simulink model "slidingSimulation"  (R2017a)
settings: Solver=VariableStepAuto  StartTime=0.0  StopTime=10.0  RelTol=1e-3
values from neighbouring files (symbols this model uses):
  leaderAcceleration = 1    [sliding.m]
undefined symbols (not defined in the file or in its folder): chi, K, Ldes, slidingFunction, wn
settings Model: Creator=tlara  LastModifiedBy=tlara

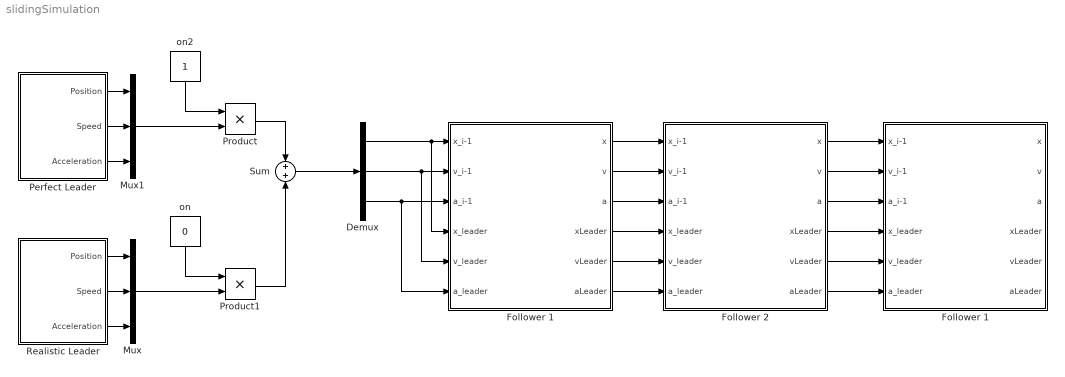
== system slidingSimulation ==
  Demux : Demux  Outputs=3
  Follower 1 : Subsystem
  "Follower 1 " : Subsystem
  Follower 2 : Subsystem
  Mux : Mux  Inputs=3
  Mux1 : Mux  Inputs=3
  Perfect Leader : Subsystem
  Product : Product
  Product1 : Product
  Realistic Leader : Subsystem
  Sum : Sum
  on : Constant  Value=0
  on2 : Constant
  wires:
  "Follower 1 "/1(x) -> Follower 2/1("x_i-1 ")
  "Follower 1 "/2(v) -> Follower 2/2(v_i-1)
  "Follower 1 "/3(a) -> Follower 2/3(a_i-1)
  "Follower 1 "/4(xLeader) -> Follower 2/4(x_leader)
  "Follower 1 "/5("vLeader ") -> Follower 2/5(v_leader)
  "Follower 1 "/6(aLeader) -> Follower 2/6(a_leader)
  Follower 2/6(aLeader) -> Follower 1/6(a_leader)
  Follower 2/5("vLeader ") -> Follower 1/5(v_leader)
  Follower 2/4(xLeader) -> Follower 1/4(x_leader)
  Follower 2/3(a) -> Follower 1/3(a_i-1)
  Follower 2/1(x) -> Follower 1/1("x_i-1 ")
  Follower 2/2(v) -> Follower 1/2(v_i-1)
  Realistic Leader/1(Position) -> Mux/1
  Realistic Leader/2(Speed) -> Mux/2
  Realistic Leader/3(Acceleration) -> Mux/3
  Perfect Leader/1(Position) -> Mux1/1
  Perfect Leader/2(Speed) -> Mux1/2
  Perfect Leader/3(Acceleration) -> Mux1/3
  Mux1/1 -> Product/2
  Mux/1 -> Product1/2
  on/1 -> Product1/1
  on2/1 -> Product/1
  Product/1 -> Sum/1
  Product1/1 -> Sum/2
  Sum/1 -> Demux/1
  Demux/3 -> "Follower 1 "/6(a_leader), "Follower 1 "/3(a_i-1)
  Demux/2 -> "Follower 1 "/5(v_leader), "Follower 1 "/2(v_i-1)
  Demux/1 -> "Follower 1 "/4(x_leader), "Follower 1 "/1("x_i-1 ")

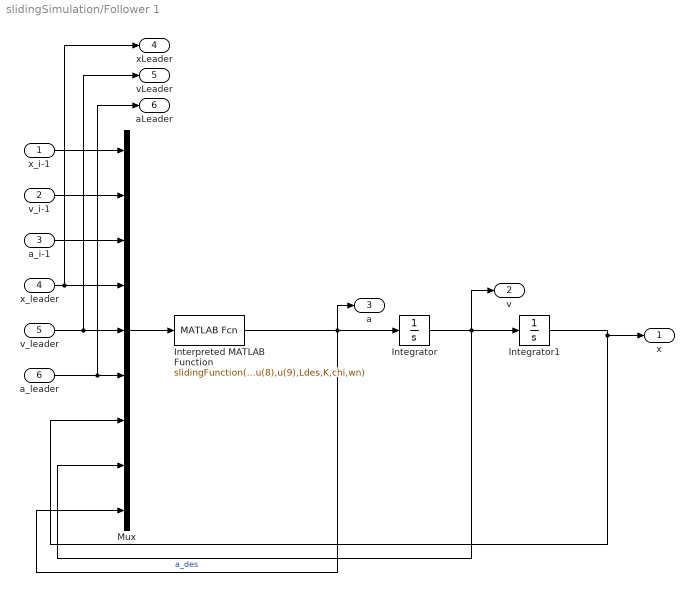
== system slidingSimulation/Follower 1 ==
  "x_i-1 " : Inport
  v_i-1 : Inport  Port=2
  a_i-1 : Inport  Port=3
  x_leader : Inport  Port=4
  v_leader : Inport  Port=5
  a_leader : Inport  Port=6
  Integrator : Integrator
  Integrator1 : Integrator
  Interpreted MATLAB Function : MATLABFcn  MATLABFcn=slidingFunction(u(1),u(2),u(3),u(4),u(5),u(6),u(7),u(8),u(9),Ldes,K,chi,wn)  OutputDimensions=1
  Mux : Mux  Inputs=9
  x : Outport
  v : Outport  Port=2
  a : Outport  Port=3
  xLeader : Outport  Port=4
  "vLeader " : Outport  Port=5
  aLeader : Outport  Port=6
  wires:
  Interpreted MATLAB Function/1 -> a/1, Mux/9, Integrator/1  "a_des"
  "x_i-1 "/1 -> Mux/1
  v_i-1/1 -> Mux/2
  a_i-1/1 -> Mux/3
  x_leader/1 -> xLeader/1, Mux/4
  v_leader/1 -> "vLeader "/1, Mux/5
  a_leader/1 -> aLeader/1, Mux/6
  Integrator1/1 -> Mux/7, x/1
  Mux/1 -> Interpreted MATLAB Function/1
  Integrator/1 -> v/1, Integrator1/1, Mux/8

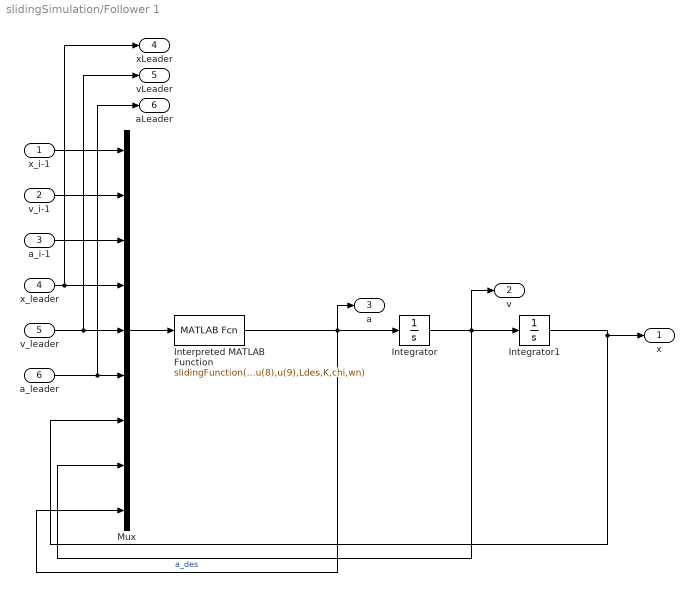
== system slidingSimulation/Follower 1  ==
  "x_i-1 " : Inport
  v_i-1 : Inport  Port=2
  a_i-1 : Inport  Port=3
  x_leader : Inport  Port=4
  v_leader : Inport  Port=5
  a_leader : Inport  Port=6
  Integrator : Integrator
  Integrator1 : Integrator
  Interpreted MATLAB Function : MATLABFcn  MATLABFcn=slidingFunction(u(1),u(2),u(3),u(4),u(5),u(6),u(7),u(8),u(9),Ldes,K,chi,wn)  OutputDimensions=1
  Mux : Mux  Inputs=9
  x : Outport
  v : Outport  Port=2
  a : Outport  Port=3
  xLeader : Outport  Port=4
  "vLeader " : Outport  Port=5
  aLeader : Outport  Port=6
  wires:
  Interpreted MATLAB Function/1 -> a/1, Mux/9, Integrator/1  "a_des"
  "x_i-1 "/1 -> Mux/1
  v_i-1/1 -> Mux/2
  a_i-1/1 -> Mux/3
  x_leader/1 -> xLeader/1, Mux/4
  v_leader/1 -> "vLeader "/1, Mux/5
  a_leader/1 -> aLeader/1, Mux/6
  Integrator1/1 -> Mux/7, x/1
  Mux/1 -> Interpreted MATLAB Function/1
  Integrator/1 -> v/1, Integrator1/1, Mux/8

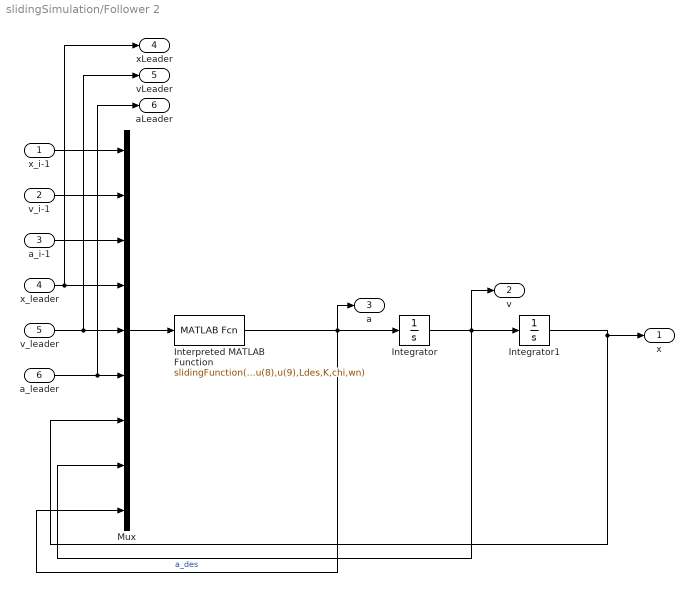
== system slidingSimulation/Follower 2 ==
  "x_i-1 " : Inport
  v_i-1 : Inport  Port=2
  a_i-1 : Inport  Port=3
  x_leader : Inport  Port=4
  v_leader : Inport  Port=5
  a_leader : Inport  Port=6
  Integrator : Integrator
  Integrator1 : Integrator
  Interpreted MATLAB Function : MATLABFcn  MATLABFcn=slidingFunction(u(1),u(2),u(3),u(4),u(5),u(6),u(7),u(8),u(9),Ldes,K,chi,wn)  OutputDimensions=1
  Mux : Mux  Inputs=9
  x : Outport
  v : Outport  Port=2
  a : Outport  Port=3
  xLeader : Outport  Port=4
  "vLeader " : Outport  Port=5
  aLeader : Outport  Port=6
  wires:
  Interpreted MATLAB Function/1 -> a/1, Mux/9, Integrator/1  "a_des"
  "x_i-1 "/1 -> Mux/1
  v_i-1/1 -> Mux/2
  a_i-1/1 -> Mux/3
  x_leader/1 -> xLeader/1, Mux/4
  v_leader/1 -> "vLeader "/1, Mux/5
  a_leader/1 -> aLeader/1, Mux/6
  Integrator1/1 -> Mux/7, x/1
  Mux/1 -> Interpreted MATLAB Function/1
  Integrator/1 -> v/1, Integrator1/1, Mux/8

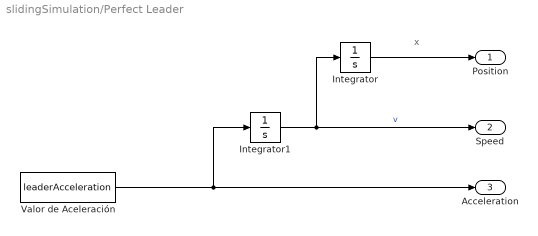
== system slidingSimulation/Perfect Leader ==
  note: x
  Integrator : Integrator
  Integrator1 : Integrator
  Valor de Aceleración : Constant  Value=leaderAcceleration
  Position : Outport
  Speed : Outport  Port=2
  Acceleration : Outport  Port=3
  wires:
  Integrator/1 -> Position/1
  Valor de Aceleración/1 -> Integrator1/1, Acceleration/1
  Integrator1/1 -> Integrator/1, Speed/1  "v"

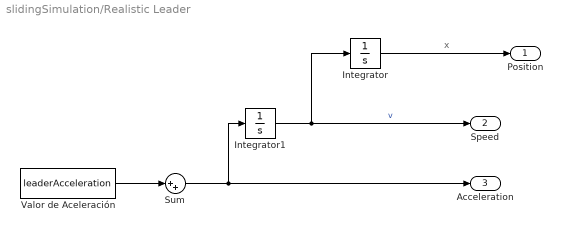
== system slidingSimulation/Realistic Leader ==
  note: x
  Integrator : Integrator
  Integrator1 : Integrator
  Sum : Sum  Inputs=|++
  Valor de Aceleración : Constant  Value=leaderAcceleration
  Position : Outport
  Speed : Outport  Port=2
  Acceleration : Outport  Port=3
  wires:
  Integrator/1 -> Position/1
  Integrator1/1 -> Integrator/1, Speed/1  "v"
  Sum/1 -> Integrator1/1, Acceleration/1
  Valor de Aceleración/1 -> Sum/1
